simulink model "f1psimu"  (R2015b)
settings: Solver=VariableStepAuto  StartTime=0.0  StopTime=5  RelTol=1e-3
settings Model: Creator=BLUE COM  LastModifiedBy=BLUE COM

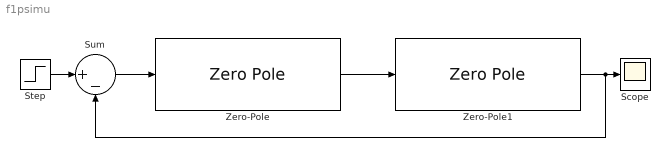
== system f1psimu ==
  Scope : Scope
  Step : Step  SampleTime=0
  Sum : Sum  Inputs=|+-
  Zero-Pole : ZeroPole  Zeros=[-1500-3122.5i -1500+3122.5i]  Poles=[0 -2.9e05]
  Zero-Pole1 : ZeroPole  Zeros=[4000]  Poles=[-1500-3122.5i -1500+3122.5i]  Gain=[-36000]
  wires:
  Step/1 -> Sum/1
  Sum/1 -> Zero-Pole/1
  Zero-Pole/1 -> Zero-Pole1/1
  Zero-Pole1/1 -> Sum/2, Scope/1
